simulink model "stellaris_fft_system"  (R2012b)
settings: Solver=FixedStepDiscrete  StartTime=0.0  StopTime=inf  FixedStep=1/1024  RelTol=1e-3
undefined symbols (not defined in the file or in its folder): get
libraries: dspsnks4 x2, dspsrcs4 x1
settings Model: Creator=peselnikmg  LastModifiedBy=peselnikmg
settings DataIOCC: SignalLoggingSaveFormat=ModelDataLogs
settings OptimizationCC: OptimizeModelRefInitCode=on  LifeSpan=1
settings HardwareCC: ProdEndianess=LittleEndian  ProdHWDeviceType=Texas Instruments->TMS470
settings RTWCC: SystemTargetFile=stellaris.tlc  TemplateMakefile=stellaris_tmf  PostCodeGenCommand=stellaris_customcode(buildInfo)  Description=TI Stellaris LaunchPad  ProcessScript=stellaris_make_rtw_hook  CodeExecutionProfiling=on  CodeProfilingSaveOptions=AllData  CodeProfilingInstrumentation=on
settings CodeAppCC: IgnoreCustomStorageClasses=off
settings STFCustomTargetCC: CodeReplacementLibrary=ANSI_C  CombineOutputUpdateFcns=on  ERTCustomFileBanners=on  SupportContinuousTime=off  SupportNonInlinedSFcns=off  GRTInterface=off  SystemTargetFile=stellaris.tlc
settings ERTTargetCC: CodeReplacementLibrary=ANSI_C  MultiwordLength=2048  ParMdlRefBuildCompliant=off  CompOptLevelCompliant=off  ConcurrentExecutionCompliant=off  ERTFirstTimeCompliant=off  ModelStepFunctionPrototypeControlCompliant=off  CPPClassGenCompliant=off  InlinedParameterPlacement=NonHierarchical  ERTCustomFileTemplate=stellaris_srmain.tlc  ConvertIfToSwitch=off  SuppressUnreachableDefaultCases=off

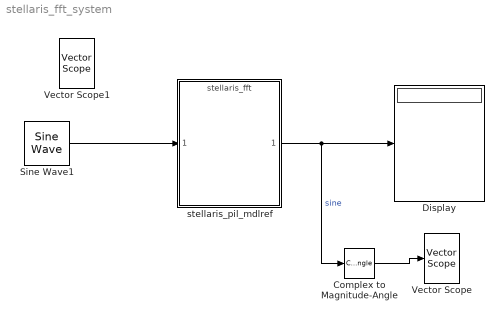
== system stellaris_fft_system ==
  Complex to Magnitude-Angle : ComplexToMagnitudeAngle  Output=Magnitude
  Display : Display
  Sine Wave1 : dspsrcs4/Sine Wave  Amplitude=1  Frequency=100  Phase=0  SampleMode=Discrete  OutComplex=Real  CompMethod=Trigonometric fcn  TableSize=Speed  SampleTime=1/1024  SamplesPerFrame=64  ResetState=Restart at time zero  dataType=single  wordLen=16  udDataType=sfix(16)  fracBitsMode=Best precision  numFracBits=15  OutDataTypeStr=single  LastOutDataTypeStr=single
  Vector Scope : dspsnks4/Vector Scope  ScopeProperties=on  Domain=Frequency  HorizSpan=1  DisplayProperties=off  AxisGrid=on  Memory=off  FrameNumber=on  AxisLegend=off  AxisZoom=off  OpenScopeAtSimStart=on  OpenScopeImmediately=off  FigPos=get(0,'defaultfigureposition')  AxisProperties=off  XUnits=Hertz  XRange=[0...Fs/2]  InheritXIncr=on  XIncr=1  XLabel=Time  XLimit=Auto  XMin=0  XMax=1  XStart=0  YUnits=dB  YLabel=Amplitude  LineProperties=off  XAxisParamsVer=6.9
      settings: YMin=-10  YMax=10
  stellaris_pil_mdlref : ModelReference  ModelNameDialog=stellaris_fft  SimulationMode=Processor-in-the-loop (PIL)  ModelReferenceVersion=1.53  CopyOfModelName=stellaris_fft  DefaultDataLogging=on
  Vector Scope1 : dspsnks4/Vector Scope  IOType=viewer  ScopeProperties=on  Domain=Time  HorizSpan=1  DisplayProperties=off  AxisGrid=on  Memory=off  FrameNumber=on  AxisLegend=off  AxisZoom=off  OpenScopeAtSimStart=on  OpenScopeImmediately=off  FigPos=get(0,'defaultfigureposition')  AxisProperties=off  XUnits=Hertz  XRange=[0...Fs/2]  InheritXIncr=on  XIncr=1  XLabel=Time  XLimit=Auto  XMin=0  XMax=1  XStart=0  YUnits=dB  YLabel=Amplitude  LineProperties=off  XAxisParamsVer=6.9
      settings: YMin=-10  YMax=10
  wires:
  stellaris_pil_mdlref/1 -> Complex to Magnitude-Angle/1, Display/1  "sine"
  Sine Wave1/1 -> stellaris_pil_mdlref/1
  Complex to Magnitude-Angle/1 -> Vector Scope/1
